simulink model "tracking_model2"  (R2017a)
settings: Solver=VariableStepAuto  StartTime=0.0  StopTime=tf  RelTol=1e-3
values from neighbouring files (symbols this model uses):
  x0 = 100    [validate_model.m]
undefined symbols (not defined in the file or in its folder): sys
settings Model: Creator=brunolnetto  LastModifiedBy=brunolnetto

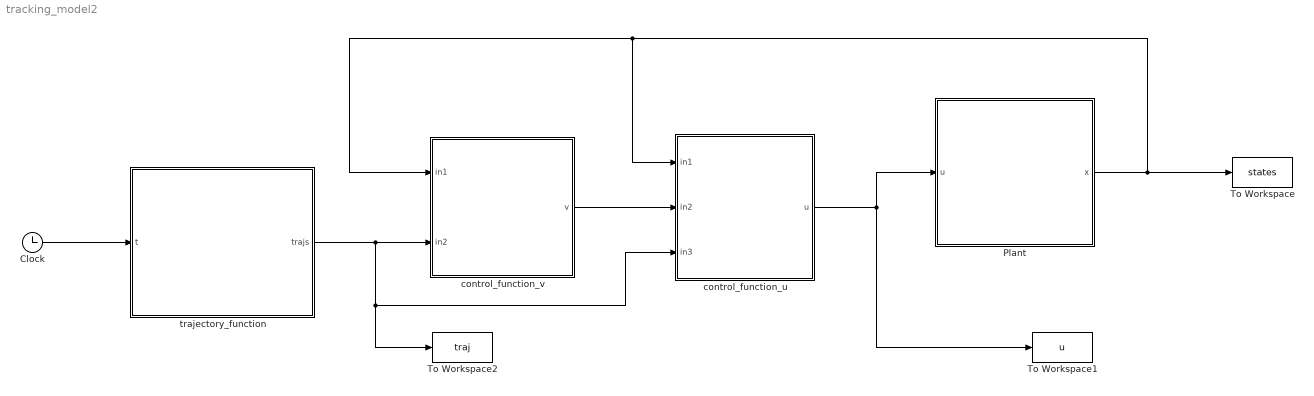
== system tracking_model2 ==
  Clock : Clock
  Plant : Subsystem
  To Workspace : ToWorkspace  VariableName=states  SaveFormat=Structure With Time  SampleTime=-1
  To Workspace1 : ToWorkspace  VariableName=u  SaveFormat=Structure With Time  SampleTime=-1
  To Workspace2 : ToWorkspace  VariableName=traj  SaveFormat=Structure With Time  SampleTime=-1
  control_function_u : MATLAB Function  TreatAsAtomicUnit=on
  control_function_v : MATLAB Function  TreatAsAtomicUnit=on
  trajectory_function : MATLAB Function  TreatAsAtomicUnit=on
  wires:
  Clock/1 -> trajectory_function/1(t)
  control_function_u/1(u) -> Plant/1(u), To Workspace1/1
  trajectory_function/1(trajs) -> control_function_u/3(in3), To Workspace2/1, control_function_v/2(in2)
  control_function_v/1(v) -> control_function_u/2(in2)
  Plant/1(x) -> control_function_u/1(in1), control_function_v/1(in1), To Workspace/1

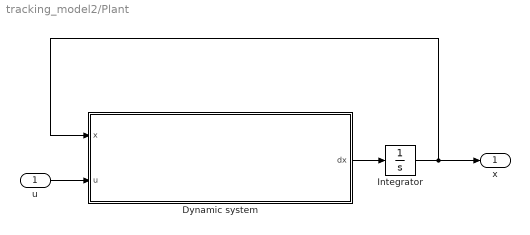
== system tracking_model2/Plant ==
  u : Inport
  Dynamic system : Subsystem
      mask Display: image('./plant.png')
  Integrator : Integrator  InitialCondition=x0
  x : Outport
  wires:
  Dynamic system/1(dx) -> Integrator/1
  u/1 -> Dynamic system/2(u)
  Integrator/1 -> x/1, Dynamic system/1(x)

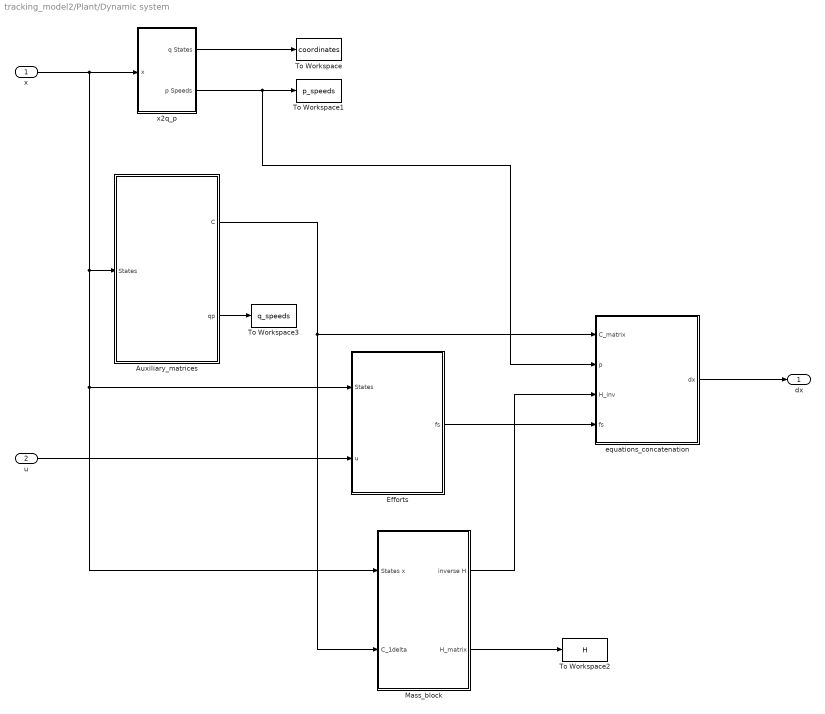
== system tracking_model2/Plant/Dynamic system ==
  x : Inport
  u : Inport  Port=2
  Auxiliary_matrices : Subsystem
  Efforts : Subsystem
  Mass_block : Subsystem
  To Workspace : ToWorkspace  VariableName=coordinates  SaveFormat=Structure With Time  SampleTime=-1
  To Workspace1 : ToWorkspace  VariableName=p_speeds  SaveFormat=Structure With Time  SampleTime=-1
  To Workspace2 : ToWorkspace  VariableName=H  SaveFormat=Structure With Time  SampleTime=-1
  To Workspace3 : ToWorkspace  VariableName=q_speeds  SaveFormat=Structure With Time  SampleTime=-1
  equations_concatenation : Subsystem
  x2q_p : Subsystem
  dx : Outport
  wires:
  Auxiliary_matrices/1(C) -> Mass_block/2("C_1delta  "), equations_concatenation/1(C_matrix)
  Auxiliary_matrices/2(qp) -> To Workspace3/1
  x2q_p/2(p Speeds) -> To Workspace1/1, equations_concatenation/2(p)
  x2q_p/1(q States) -> To Workspace/1
  Efforts/1(fs) -> equations_concatenation/4(fs)
  Mass_block/1(inverse H) -> equations_concatenation/3(H_inv)
  equations_concatenation/1(dx) -> dx/1
  u/1 -> Efforts/2(u)
  x/1 -> x2q_p/1(x), Efforts/1(States), Mass_block/1(States x), Auxiliary_matrices/1(States)
  Mass_block/2(H_matrix) -> To Workspace2/1

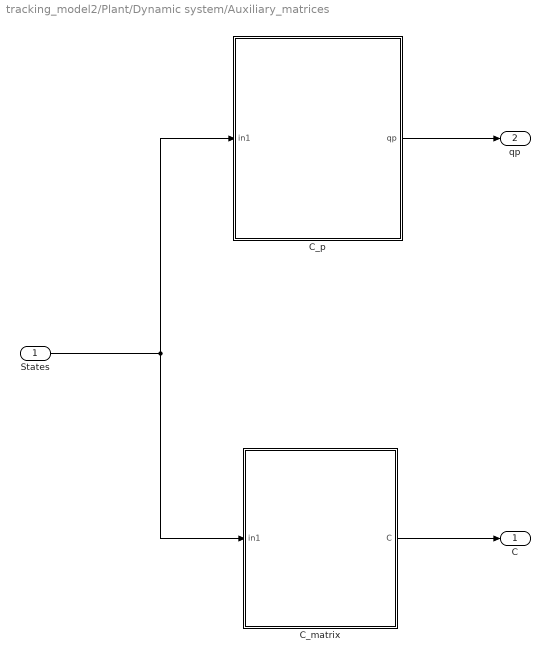
== system tracking_model2/Plant/Dynamic system/Auxiliary_matrices ==
  States : Inport
  C_matrix : MATLAB Function  TreatAsAtomicUnit=on
  C_p : MATLAB Function  TreatAsAtomicUnit=on
  C : Outport
  qp : Outport  Port=2
  wires:
  C_matrix/1(C) -> C/1
  States/1 -> C_p/1(in1), C_matrix/1(in1)
  C_p/1(qp) -> qp/1

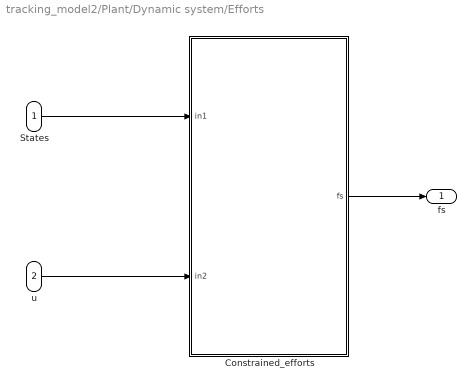
== system tracking_model2/Plant/Dynamic system/Efforts ==
  States : Inport
  u : Inport  Port=2
  Constrained_efforts : MATLAB Function  TreatAsAtomicUnit=on
  fs : Outport
  wires:
  States/1 -> Constrained_efforts/1(in1)
  u/1 -> Constrained_efforts/2(in2)
  Constrained_efforts/1(fs) -> fs/1

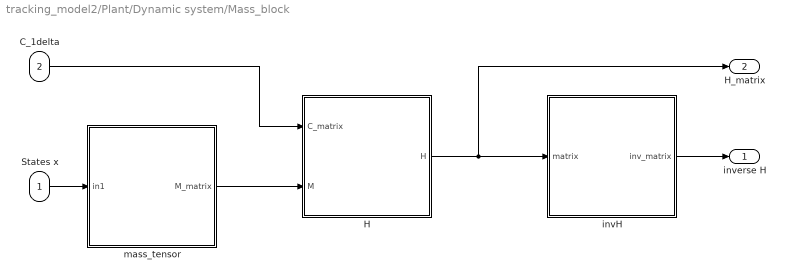
== system tracking_model2/Plant/Dynamic system/Mass_block ==
  States x : Inport
  "C_1delta  " : Inport  Port=2
  H : MATLAB Function  TreatAsAtomicUnit=on
  invH : MATLAB Function  TreatAsAtomicUnit=on
  mass_tensor : MATLAB Function  TreatAsAtomicUnit=on
  inverse H : Outport
  H_matrix : Outport  Port=2
  wires:
  States x/1 -> mass_tensor/1(in1)
  "C_1delta  "/1 -> H/1(C_matrix)
  invH/1(inv_matrix) -> inverse H/1
  H/1(H) -> invH/1(matrix), H_matrix/1
  mass_tensor/1(M_matrix) -> H/2(M)

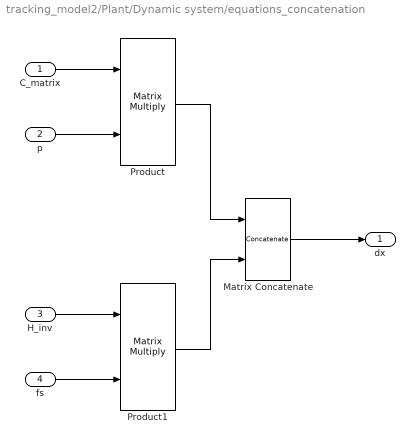
== system tracking_model2/Plant/Dynamic system/equations_concatenation ==
  C_matrix : Inport
  p : Inport  Port=2
  H_inv : Inport  Port=3
  fs : Inport  Port=4
  Matrix Concatenate : Concatenate  ConcatenateDimension=2
  Product : Product  Multiplication=Matrix(*)
  Product1 : Product  Multiplication=Matrix(*)
  dx : Outport
  wires:
  Product/1 -> Matrix Concatenate/1
  p/1 -> Product/2
  C_matrix/1 -> Product/1
  Product1/1 -> Matrix Concatenate/2
  H_inv/1 -> Product1/1
  fs/1 -> Product1/2
  Matrix Concatenate/1 -> dx/1

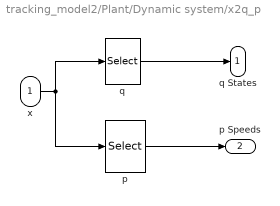
== system tracking_model2/Plant/Dynamic system/x2q_p ==
  x : Inport
  p : Selector  InputPortWidth=length(sys.kin.q) + length(sys.kin.p{end})  IndexOptions=Index vector (dialog)  Indices=(length(sys.kin.q))+1:(length(sys.kin.q) + length(sys.kin.p{end}))  OutputSizes=1
  q : Selector  InputPortWidth=length(sys.kin.q) + length(sys.kin.p{end})  IndexOptions=Index vector (dialog)  Indices=1:length(sys.kin.q)  OutputSizes=1
  q States : Outport
  p Speeds : Outport  Port=2
  wires:
  x/1 -> p/1, q/1
  q/1 -> q States/1
  p/1 -> p Speeds/1

== matlab function tracking_model2/control_function_v ==
  data: in1 input; v output; in2 input
function v = ControlFunction(in1,in2)

%    This function was generated by the Symbolic Math Toolbox version 7.2.

%    11-Jan-2021 14:43:12



p1 = in1(7,:);

p2 = in1(8,:);

p3 = in1(9,:);

th = in1(3,:);

x = in1(1,:);

y = in1(2,:);

y1_ref = in2(1,:);

y2_ref = in2(4,:);

y3_ref = in2(7,:);

yp1_ref = in2(2,:);

yp2_ref = in2(5,:);

yp3_ref = in2(8,:);

v = [p1.*-3.438624078545841-p2.*2.652700203337989-p3.*3.377020513851819e-15-th.*1.00163037277543e-14-x.*6.884313755249821-y.*1.038824780522046e1+y1_ref.*6.884313755249821+y2_ref.*1.038824780522046e1+y3_ref.*1.00163037277543e-14+yp1_ref.*3.438624078545841+yp2_ref.*2.652700203337989+yp3_ref.*3.377020513851819e-15;0.0;0.0;p1.*-2.652700278465205-p2.*7.736290108681494-p3.*1.635524904530068e-15-th.*1.056093842869619e-14-x.*1.038824829359606e1-y.*2.371441739383425e1+y1_ref.*1.038824829359606e1+y2_ref.*2.371441739383425e1+y3_ref.*1.056093842869619e-14+yp1_ref.*2.652700278465205+yp2_ref.*7.736290108681494+yp3_ref.*1.635524904530068e-15;0.0;0.0;p1.*-5.380262330691395e-15-p2.*4.786557594007766e-16-p3.*4.177097391684711-th.*6.652662314872519-x.*1.163926222557845e-14-y.*9.477276537930718e-15+y1_ref.*1.163926222557845e-14+y2_ref.*9.477276537930718e-15+y3_ref.*6.652662314872519+yp1_ref.*5.380262330691395e-15+yp2_ref.*4.786557594007766e-16+yp3_ref.*4.177097391684711;0.0;0.0];

end

== matlab function tracking_model2/Plant/Dynamic system/Mass_block/mass_tensor ==
  data: in1 input; M_matrix output
function M_matrix = Mass_matrix(in1)

%    This function was generated by the Symbolic Math Toolbox version 7.2.

%    11-Jan-2021 14:43:15



th = in1(3,:);

th1 = in1(4,:);

th2 = in1(5,:);

th3 = in1(6,:);

t2 = cos(th);

t3 = cos(th1);

t4 = cos(th2);

t5 = cos(th3);

t6 = sin(th);

t8 = t2.*(1.0./8.0);

t9 = sqrt(3.0);

t10 = t6.*t9.*(1.0./8.0);

t7 = t8-t10;

t11 = t8+t10;

t13 = t6.*(1.0./8.0);

t14 = t2.*t9.*(1.0./8.0);

t12 = t13-t14;

t15 = t13+t14;

M_matrix = reshape([2.11e2./5.0e2,0.0,0.0,0.0,0.0,0.0,0.0,2.11e2./5.0e2,0.0,0.0,0.0,0.0,0.0,0.0,t2.^2.*4.625e-3+t3.^2.*2.518133623269337e-7+t4.^2.*2.518133623269337e-7+t5.^2.*2.518133623269337e-7+t6.^2.*4.625e-3+t7.^2.*(3.7e1./5.0e2)+t11.^2.*(3.7e1./5.0e2)+t12.^2.*(3.7e1./5.0e2)+t15.^2.*(3.7e1./5.0e2)+2.520833333333333e-4,0.0,0.0,0.0,0.0,0.0,0.0,0.0,0.0,0.0,0.0,0.0,0.0,0.0,0.0,0.0,0.0,0.0,0.0,0.0,0.0,0.0],[6,6]);

end

== matlab function tracking_model2/Plant/Dynamic system/Auxiliary_matrices/C_matrix ==
  data: in1 input; C output
function C = ConstraintMatrix(in1)

%    This function was generated by the Symbolic Math Toolbox version 7.2.

%    11-Jan-2021 14:43:14



th = in1(3,:);

t2 = pi.*(1.0./3.0);

t3 = t2+th;

C = reshape([1.0,0.0,0.0,sin(th).*(5.0e2./4.3e1),cos(th+pi.*(1.0./6.0)).*(5.0e2./4.3e1),sin(t3).*(-5.0e2./4.3e1),0.0,1.0,0.0,cos(th).*(-5.0e2./4.3e1),cos(th-pi.*(1.0./3.0)).*(5.0e2./4.3e1),cos(t3).*(5.0e2./4.3e1),0.0,0.0,1.0,-1.25e2./4.3e1,-1.25e2./4.3e1,-1.25e2./4.3e1],[6,3]);

end

== matlab function tracking_model2/trajectory_function ==
  data: t input; trajs output
function trajs = TrajectoryGenerator(t)

%    This function was generated by the Symbolic Math Toolbox version 7.2.

%    11-Jan-2021 14:43:13



t2 = cos(t);

t3 = sin(t);

trajs = [t2;-t3;-t2;t3;t2;-t3;t;1.0;0.0];

end

== matlab function tracking_model2/control_function_u ==
  data: in1 input; u output; in2 input; in3 input
function u = ControlFunction(in1,in2,in3)

%    This function was generated by the Symbolic Math Toolbox version 7.2.

%    11-Jan-2021 14:43:10



p1 = in1(7,:);

p2 = in1(8,:);

p3 = in1(9,:);

th = in1(3,:);

th1 = in1(4,:);

th2 = in1(5,:);

th3 = in1(6,:);

v1 = in2(1,:);

x = in1(1,:);

y = in1(2,:);

y1_ref = in3(1,:);

y2_ref = in3(4,:);

y3_ref = in3(7,:);

yp1_ref = in3(2,:);

yp2_ref = in3(5,:);

yp3_ref = in3(8,:);

ypp1_ref = in3(3,:);

ypp2_ref = in3(6,:);

ypp3_ref = in3(9,:);

t2 = sin(th);

t3 = cos(th);

t4 = t2.^2;

t5 = t3.^2;

t6 = t5.*5.585863854409629e-2;

t7 = t4.*5.585863854409629e-2;

t8 = t6+t7;

t9 = 1.0./t8;

t10 = t5.*2.234345541763852e-1;

t11 = t4.*2.234345541763852e-1;

t12 = t10+t11;

t13 = 1.0./t12;

t14 = cos(th1);

t15 = cos(th2);

t16 = cos(th3);

t17 = t14.^2;

t18 = t15.^2;

t19 = t16.^2;

t20 = p3.^2;

t21 = t5.*5.836328869266157e-6;

t22 = t4.*5.836328869266157e-6;

t23 = t5.*t17.*1.040317779359265e-10;

t24 = t5.*t18.*1.040317779359265e-10;

t25 = t5.*t19.*1.040317779359265e-10;

t26 = t4.*t17.*1.040317779359265e-10;

t27 = t4.*t18.*1.040317779359265e-10;

t28 = t4.*t19.*1.040317779359265e-10;

t29 = t21+t22+t23+t24+t25+t26+t27+t28;

t30 = 1.0./t29;

t31 = sin(th1);

t32 = sin(th2);

t33 = sin(th3);

t34 = t31.^2;

t35 = t32.^2;

t36 = t33.^2;

t37 = th1.*2.0;

t38 = sin(t37);

t39 = th2.*2.0;

t40 = sin(t39);

t41 = th3.*2.0;

t42 = sin(t41);

t43 = t5.*1.394728536509132e-3;

t44 = t4.*1.394728536509132e-3;

t45 = t43+t44;

t46 = 1.0./t45;

t47 = p1.*p3.*t3.*t5.*t15.*t30.*t32.*t35.*-6.049843728929489e-17;

t48 = p1.*p3.*t3.*t5.*t16.*t30.*t33.*t36.*6.049843728929489e-17;

t49 = p2.*p3.*t2.*t4.*t15.*t30.*t32.*t35.*-6.049843728929489e-17;

t50 = p2.*p3.*t2.*t4.*t16.*t30.*t33.*t36.*6.049843728929489e-17;

t51 = p1.*p3.*t3.*t4.*t15.*t30.*t32.*t35.*-6.049843728929489e-17;

t52 = p1.*p3.*t3.*t5.*t15.*t30.*t32.*t34.*-6.049843728929489e-17;

t53 = p2.*p3.*t2.*t5.*t15.*t30.*t32.*t35.*-6.049843728929489e-17;

t54 = p1.*p3.*t3.*t4.*t16.*t30.*t33.*t36.*6.049843728929489e-17;

t55 = p1.*p3.*t3.*t5.*t15.*t30.*t32.*t36.*-6.049843728929489e-17;

t56 = p1.*p3.*t3.*t5.*t16.*t30.*t33.*t34.*6.049843728929489e-17;

t57 = p2.*p3.*t2.*t5.*t16.*t30.*t33.*t36.*6.049843728929489e-17;

t58 = p1.*p3.*t3.*t5.*t16.*t30.*t33.*t35.*6.049843728929489e-17;

t59 = p2.*p3.*t2.*t4.*t15.*t30.*t32.*t34.*-6.049843728929489e-17;

t60 = p2.*p3.*t2.*t4.*t15.*t30.*t32.*t36.*-6.049843728929489e-17;

t61 = p2.*p3.*t2.*t4.*t16.*t30.*t33.*t34.*6.049843728929489e-17;

t62 = p2.*p3.*t2.*t4.*t16.*t30.*t33.*t35.*6.049843728929489e-17;

t63 = p1.*p3.*t3.*t4.*t15.*t30.*t32.*t34.*-6.049843728929489e-17;

t64 = p2.*p3.*t2.*t5.*t15.*t30.*t32.*t34.*-6.049843728929489e-17;

t65 = p1.*p3.*t3.*t4.*t15.*t30.*t32.*t36.*-6.049843728929489e-17;

t66 = p1.*p3.*t3.*t4.*t16.*t30.*t33.*t34.*6.049843728929489e-17;

t67 = p1.*p3.*t3.*t4.*t16.*t30.*t33.*t35.*6.049843728929489e-17;

t68 = p2.*p3.*t2.*t5.*t15.*t30.*t32.*t36.*-6.049843728929489e-17;

t69 = p2.*p3.*t2.*t5.*t16.*t30.*t33.*t34.*6.049843728929489e-17;

t70 = p2.*p3.*t2.*t5.*t16.*t30.*t33.*t35.*6.049843728929489e-17;

t71 = p2.*t3.*t13.*-1.081184912022583e-2;

t72 = t3.*t13.*y.*-1.081184912022583e-2;

t73 = t3.*t13.*y2_ref.*1.081184912022583e-2;

t74 = t3.*t13.*yp2_ref.*1.081184912022583e-2;

t75 = t3.*t13.*ypp2_ref.*2.702962280056457e-3;

t76 = p1.*t2.*t13.*1.081184912022583e-2;

t77 = t2.*t13.*x.*1.081184912022583e-2;

t78 = t2.*t13.*y1_ref.*-1.081184912022583e-2;

t79 = t2.*t13.*yp1_ref.*-1.081184912022583e-2;

t80 = t2.*t13.*ypp1_ref.*-2.702962280056457e-3;

t81 = t5.*t20.*t30.*t34.*1.013340774614903e-53;

t82 = t5.*t20.*t30.*t35.*1.013340774614903e-53;

t83 = t5.*t20.*t30.*t36.*1.013340774614903e-53;

t84 = p3.*t5.*t9.*t34.*-6.451583127809397e-9;

t85 = p3.*t5.*t9.*t35.*-6.451583127809397e-9;

t86 = p3.*t5.*t9.*t36.*-6.451583127809397e-9;

t87 = t4.*t20.*t30.*t34.*1.013340774614903e-53;

t88 = t4.*t20.*t30.*t35.*1.013340774614903e-53;

t89 = t4.*t20.*t30.*t36.*1.013340774614903e-53;

t90 = t5.*t9.*t34.*th.*-6.451583127809397e-9;

t91 = t5.*t9.*t35.*th.*-6.451583127809397e-9;

t92 = t5.*t9.*t36.*th.*-6.451583127809397e-9;

t93 = t5.*t9.*t34.*v1.*1.612895781952349e-9;

t94 = t5.*t9.*t35.*v1.*1.612895781952349e-9;

t95 = t5.*t9.*t36.*v1.*1.612895781952349e-9;

t96 = t5.*t9.*t34.*y3_ref.*6.451583127809397e-9;

t97 = t5.*t9.*t35.*y3_ref.*6.451583127809397e-9;

t98 = t5.*t9.*t36.*y3_ref.*6.451583127809397e-9;

t99 = t5.*t9.*t34.*yp3_ref.*6.451583127809397e-9;

t100 = t5.*t9.*t35.*yp3_ref.*6.451583127809397e-9;

t101 = t5.*t9.*t36.*yp3_ref.*6.451583127809397e-9;

t102 = t5.*t9.*t34.*ypp3_ref.*1.612895781952349e-9;

t103 = t5.*t9.*t35.*ypp3_ref.*1.612895781952349e-9;

t104 = t5.*t9.*t36.*ypp3_ref.*1.612895781952349e-9;

t105 = p3.*t4.*t9.*t34.*-6.451583127809397e-9;

t106 = p3.*t4.*t9.*t35.*-6.451583127809397e-9;

t107 = p3.*t4.*t9.*t36.*-6.451583127809397e-9;

t108 = t4.*t9.*t34.*th.*-6.451583127809397e-9;

t109 = t4.*t9.*t35.*th.*-6.451583127809397e-9;

t110 = t4.*t9.*t36.*th.*-6.451583127809397e-9;

t111 = t4.*t9.*t34.*v1.*1.612895781952349e-9;

t112 = t4.*t9.*t35.*v1.*1.612895781952349e-9;

t113 = t4.*t9.*t36.*v1.*1.612895781952349e-9;

t114 = t4.*t9.*t34.*y3_ref.*6.451583127809397e-9;

t115 = t4.*t9.*t35.*y3_ref.*6.451583127809397e-9;

t116 = t4.*t9.*t36.*y3_ref.*6.451583127809397e-9;

t117 = t4.*t9.*t34.*yp3_ref.*6.451583127809397e-9;

t118 = t4.*t9.*t35.*yp3_ref.*6.451583127809397e-9;

t119 = t4.*t9.*t36.*yp3_ref.*6.451583127809397e-9;

t120 = t4.*t9.*t34.*ypp3_ref.*1.612895781952349e-9;

t121 = t4.*t9.*t35.*ypp3_ref.*1.612895781952349e-9;

t122 = t4.*t9.*t36.*ypp3_ref.*1.612895781952349e-9;

t123 = t5.*t20.*t30.*t38.*-2.449573643318391e-13;

t124 = t5.*t20.*t30.*t40.*-2.449573643318391e-13;

t125 = t5.*t20.*t30.*t42.*-2.449573643318391e-13;

t126 = t4.*t20.*t30.*t38.*-2.449573643318391e-13;

t127 = t4.*t20.*t30.*t40.*-2.449573643318391e-13;

t128 = t4.*t20.*t30.*t42.*-2.449573643318391e-13;

t129 = t5.*t20.*t30.*t34.*t38.*4.366098631815762e-18;

t130 = t5.*t20.*t30.*t35.*t38.*4.366098631815762e-18;

t131 = t5.*t20.*t30.*t34.*t40.*4.366098631815762e-18;

t132 = t5.*t20.*t30.*t36.*t38.*4.366098631815762e-18;

t133 = t5.*t20.*t30.*t35.*t40.*4.366098631815762e-18;

t134 = t5.*t20.*t30.*t34.*t42.*4.366098631815762e-18;

t135 = t5.*t20.*t30.*t36.*t40.*4.366098631815762e-18;

t136 = t5.*t20.*t30.*t35.*t42.*4.366098631815762e-18;

t137 = t5.*t20.*t30.*t36.*t42.*4.366098631815762e-18;

t138 = t4.*t20.*t30.*t34.*t38.*4.366098631815762e-18;

t139 = t4.*t20.*t30.*t35.*t38.*4.366098631815762e-18;

t140 = t4.*t20.*t30.*t34.*t40.*4.366098631815762e-18;

t141 = t4.*t20.*t30.*t36.*t38.*4.366098631815762e-18;

t142 = t4.*t20.*t30.*t35.*t40.*4.366098631815762e-18;

t143 = t4.*t20.*t30.*t34.*t42.*4.366098631815762e-18;

t144 = t4.*t20.*t30.*t36.*t40.*4.366098631815762e-18;

t145 = t4.*t20.*t30.*t35.*t42.*4.366098631815762e-18;

t146 = t4.*t20.*t30.*t36.*t42.*4.366098631815762e-18;

t147 = p2.*p3.*t3.*t5.*t14.*t30.*t31.*t34.*6.98575781090522e-17;

t148 = p2.*p3.*t3.*t5.*t15.*t30.*t32.*t35.*-3.49287890545261e-17;

t149 = p2.*p3.*t3.*t5.*t16.*t30.*t33.*t36.*-3.49287890545261e-17;

t150 = p1.*p3.*t2.*t4.*t14.*t30.*t31.*t34.*-6.98575781090522e-17;

t151 = p1.*p3.*t2.*t4.*t15.*t30.*t32.*t35.*3.49287890545261e-17;

t152 = p1.*p3.*t2.*t4.*t16.*t30.*t33.*t36.*3.49287890545261e-17;

t153 = p2.*p3.*t3.*t5.*t14.*t30.*t31.*-3.919317829309426e-12;

t154 = p1.*p3.*t3.*t5.*t15.*t30.*t32.*3.394228805687245e-12;

t155 = p2.*p3.*t3.*t5.*t15.*t30.*t32.*1.959658914654713e-12;

t156 = p1.*p3.*t3.*t5.*t16.*t30.*t33.*-3.394228805687245e-12;

t157 = p2.*p3.*t3.*t5.*t16.*t30.*t33.*1.959658914654713e-12;

t158 = p1.*p3.*t2.*t4.*t14.*t30.*t31.*3.919317829309426e-12;

t159 = p1.*p3.*t2.*t4.*t15.*t30.*t32.*-1.959658914654713e-12;

t160 = p2.*p3.*t2.*t4.*t15.*t30.*t32.*3.394228805687245e-12;

t161 = p1.*p3.*t2.*t4.*t16.*t30.*t33.*-1.959658914654713e-12;

t162 = p2.*p3.*t2.*t4.*t16.*t30.*t33.*-3.394228805687245e-12;

t163 = p1.*p3.*t2.*t5.*t14.*t30.*t31.*3.919317829309426e-12;

t164 = p2.*p3.*t3.*t4.*t14.*t30.*t31.*-3.919317829309426e-12;

t165 = p1.*p3.*t3.*t4.*t15.*t30.*t32.*3.394228805687245e-12;

t166 = p1.*p3.*t2.*t5.*t15.*t30.*t32.*-1.959658914654713e-12;

t167 = p2.*p3.*t3.*t4.*t15.*t30.*t32.*1.959658914654713e-12;

t168 = p2.*p3.*t2.*t5.*t15.*t30.*t32.*3.394228805687245e-12;

t169 = p1.*p3.*t3.*t4.*t16.*t30.*t33.*-3.394228805687245e-12;

t170 = p1.*p3.*t2.*t5.*t16.*t30.*t33.*-1.959658914654713e-12;

t171 = p2.*p3.*t3.*t4.*t16.*t30.*t33.*1.959658914654713e-12;

t172 = p2.*p3.*t2.*t5.*t16.*t30.*t33.*-3.394228805687245e-12;

t173 = p1.*p3.*t2.*t5.*t14.*t30.*t31.*t34.*-6.98575781090522e-17;

t174 = p2.*p3.*t3.*t4.*t14.*t30.*t31.*t34.*6.98575781090522e-17;

t175 = p1.*p3.*t2.*t5.*t15.*t30.*t32.*t35.*3.49287890545261e-17;

t176 = p2.*p3.*t3.*t4.*t15.*t30.*t32.*t35.*-3.49287890545261e-17;

t177 = p2.*p3.*t3.*t5.*t14.*t30.*t31.*t35.*6.98575781090522e-17;

t178 = p1.*p3.*t2.*t5.*t16.*t30.*t33.*t36.*3.49287890545261e-17;

t179 = p2.*p3.*t3.*t5.*t14.*t30.*t31.*t36.*6.98575781090522e-17;

t180 = p2.*p3.*t3.*t5.*t15.*t30.*t32.*t34.*-3.49287890545261e-17;

t181 = p2.*p3.*t3.*t4.*t16.*t30.*t33.*t36.*-3.49287890545261e-17;

t182 = p2.*p3.*t3.*t5.*t15.*t30.*t32.*t36.*-3.49287890545261e-17;

t183 = p2.*p3.*t3.*t5.*t16.*t30.*t33.*t34.*-3.49287890545261e-17;

t184 = p2.*p3.*t3.*t5.*t16.*t30.*t33.*t35.*-3.49287890545261e-17;

t185 = p1.*p3.*t2.*t4.*t14.*t30.*t31.*t35.*-6.98575781090522e-17;

t186 = p1.*p3.*t2.*t4.*t14.*t30.*t31.*t36.*-6.98575781090522e-17;

t187 = p1.*p3.*t2.*t4.*t15.*t30.*t32.*t34.*3.49287890545261e-17;

t188 = p1.*p3.*t2.*t4.*t15.*t30.*t32.*t36.*3.49287890545261e-17;

t189 = p1.*p3.*t2.*t4.*t16.*t30.*t33.*t34.*3.49287890545261e-17;

t190 = p1.*p3.*t2.*t4.*t16.*t30.*t33.*t35.*3.49287890545261e-17;

t191 = p1.*p3.*t2.*t5.*t14.*t30.*t31.*t35.*-6.98575781090522e-17;

t192 = p1.*p3.*t2.*t5.*t14.*t30.*t31.*t36.*-6.98575781090522e-17;

t193 = p1.*p3.*t2.*t5.*t15.*t30.*t32.*t34.*3.49287890545261e-17;

t194 = p2.*p3.*t3.*t4.*t14.*t30.*t31.*t35.*6.98575781090522e-17;

t195 = p2.*p3.*t3.*t4.*t14.*t30.*t31.*t36.*6.98575781090522e-17;

t196 = p2.*p3.*t3.*t4.*t15.*t30.*t32.*t34.*-3.49287890545261e-17;

t197 = p1.*p3.*t2.*t5.*t15.*t30.*t32.*t36.*3.49287890545261e-17;

t198 = p1.*p3.*t2.*t5.*t16.*t30.*t33.*t34.*3.49287890545261e-17;

t199 = p1.*p3.*t2.*t5.*t16.*t30.*t33.*t35.*3.49287890545261e-17;

t200 = p2.*p3.*t3.*t4.*t15.*t30.*t32.*t36.*-3.49287890545261e-17;

t201 = p2.*p3.*t3.*t4.*t16.*t30.*t33.*t34.*-3.49287890545261e-17;

t202 = p2.*p3.*t3.*t4.*t16.*t30.*t33.*t35.*-3.49287890545261e-17;

u = [t47+t48+t49+t50+t51+t52+t53+t54+t55+t56+t57+t58+t59+t60+t61+t62+t63+t64+t65+t66+t67+t68+t69+t70+t81+t82+t83+t84+t85+t86+t87+t88+t89+t90+t91+t92+t93+t94+t95+t96+t97+t98+t99+t100+t101+t102+t103+t104+t105+t106+t107+t108+t109+t110+t111+t112+t113+t114+t115+t116+t117+t118+t119+t120+t121+t122+t129+t130+t131+t132+t133+t134+t135+t136+t137+t138+t139+t140+t141+t142+t143+t144+t145+t146+t147+t148+t149+t150+t151+t152+t173+t174+t175+t176+t177+t178+t179+t180+t181+t182+t183+t184+t185+t186+t187+t188+t189+t190+t191+t192+t193+t194+t195+t196+t197+t198+t199+t200+t201+t202-p1.*t2.*t13.*2.162369824045165e-2+p3.*t4.*t9.*3.619622303627885e-4-p1.*t3.*t13.*5.732577381693205e-42-p2.*t2.*t13.*5.732577381693205e-42+p3.*t5.*t9.*3.619622303627885e-4+p2.*t3.*t13.*2.162369824045165e-2-t4.*t20.*t30.*5.685288085588199e-49-t5.*t20.*t30.*5.685288085588199e-49+t4.*t9.*th.*3.619622303627885e-4+t5.*t9.*th.*3.619622303627885e-4-t4.*t9.*v1.*9.049055759069713e-5-t5.*t9.*v1.*9.049055759069713e-5+t2.*t13.*v1.*5.405924560112914e-3-t3.*t13.*v1.*5.405924560112914e-3-t2.*t13.*x.*2.162369824045165e-2-t3.*t13.*x.*5.732577381693205e-42-t2.*t13.*y.*5.732577381693205e-42+t3.*t13.*y.*2.162369824045165e-2+t2.*t13.*y1_ref.*2.162369824045165e-2-t4.*t9.*y3_ref.*3.619622303627885e-4+t2.*t13.*y2_ref.*5.732577381693205e-42+t3.*t13.*y1_ref.*5.732577381693205e-42-t5.*t9.*y3_ref.*3.619622303627885e-4-t3.*t13.*y2_ref.*2.162369824045165e-2+t2.*t13.*yp1_ref.*2.162369824045165e-2-t4.*t9.*yp3_ref.*3.619622303627885e-4+t2.*t13.*yp2_ref.*5.732577381693205e-42+t3.*t13.*yp1_ref.*5.732577381693205e-42-t5.*t9.*yp3_ref.*3.619622303627885e-4-t3.*t13.*yp2_ref.*2.162369824045165e-2+t2.*t13.*ypp1_ref.*5.405924560112914e-3-t4.*t9.*ypp3_ref.*9.049055759069713e-5+t2.*t13.*ypp2_ref.*1.433144345423301e-42+t3.*t13.*ypp1_ref.*1.433144345423301e-42-t5.*t9.*ypp3_ref.*9.049055759069713e-5-t3.*t13.*ypp2_ref.*5.405924560112914e-3-t4.*t20.*t30.*t38.*2.449573643318391e-13-t5.*t20.*t30.*t38.*2.449573643318391e-13-t4.*t20.*t30.*t40.*2.449573643318391e-13-t5.*t20.*t30.*t40.*2.449573643318391e-13-t4.*t20.*t30.*t42.*2.449573643318391e-13-t5.*t20.*t30.*t42.*2.449573643318391e-13+t4.*t14.*t20.*t31.*t46.*2.341408548744586e-10+t5.*t14.*t20.*t31.*t46.*2.341408548744586e-10-t4.*t15.*t20.*t32.*t46.*1.170704274372293e-10-t5.*t15.*t20.*t32.*t46.*1.170704274372293e-10-t4.*t16.*t20.*t33.*t46.*1.170704274372293e-10-t5.*t16.*t20.*t33.*t46.*1.170704274372293e-10+p1.*p3.*t2.*t4.*t14.*t30.*t31.*3.919317829309426e-12+p1.*p3.*t2.*t5.*t14.*t30.*t31.*3.919317829309426e-12-p1.*p3.*t2.*t4.*t15.*t30.*t32.*1.959658914654713e-12-p2.*p3.*t3.*t4.*t14.*t30.*t31.*3.919317829309426e-12-p1.*p3.*t2.*t5.*t15.*t30.*t32.*1.959658914654713e-12+p1.*p3.*t3.*t4.*t15.*t30.*t32.*3.394228805687245e-12+p2.*p3.*t2.*t4.*t15.*t30.*t32.*3.394228805687245e-12-p2.*p3.*t3.*t5.*t14.*t30.*t31.*3.919317829309426e-12-p1.*p3.*t2.*t4.*t16.*t30.*t33.*1.959658914654713e-12+p1.*p3.*t3.*t5.*t15.*t30.*t32.*3.394228805687245e-12+p2.*p3.*t2.*t5.*t15.*t30.*t32.*3.394228805687245e-12+p2.*p3.*t3.*t4.*t15.*t30.*t32.*1.959658914654713e-12-p1.*p3.*t2.*t5.*t16.*t30.*t33.*1.959658914654713e-12-p1.*p3.*t3.*t4.*t16.*t30.*t33.*3.394228805687245e-12-p2.*p3.*t2.*t4.*t16.*t30.*t33.*3.394228805687245e-12+p2.*p3.*t3.*t5.*t15.*t30.*t32.*1.959658914654713e-12-p1.*p3.*t3.*t5.*t16.*t30.*t33.*3.394228805687245e-12-p2.*p3.*t2.*t5.*t16.*t30.*t33.*3.394228805687245e-12+p2.*p3.*t3.*t4.*t16.*t30.*t33.*1.959658914654713e-12+p2.*p3.*t3.*t5.*t16.*t30.*t33.*1.959658914654713e-12;t47+t48+t49+t50+t51+t52+t53+t54+t55+t56+t57+t58+t59+t60+t61+t62+t63+t64+t65+t66+t67+t68+t69+t70+t71+t72+t73+t74+t75+t76+t77+t78+t79+t80+t123+t124+t125+t126+t127+t128+t153+t154+t155+t156+t157+t158+t159+t160+t161+t162+t163+t164+t165+t166+t167+t168+t169+t170+t171+t172+p3.*t4.*t9.*3.619622303627885e-4-p1.*t3.*t13.*1.8726672e-2-p2.*t2.*t13.*1.8726672e-2+p3.*t5.*t9.*3.619622303627885e-4-t4.*t20.*t30.*5.685288085588199e-49-t5.*t20.*t30.*5.685288085588199e-49+t4.*t9.*th.*3.619622303627885e-4+t5.*t9.*th.*3.619622303627885e-4-t4.*t9.*v1.*9.049055759069713e-5-t5.*t9.*v1.*9.049055759069713e-5+t2.*t13.*v1.*1.978705719943543e-3+t3.*t13.*v1.*7.384630280056457e-3-t3.*t13.*x.*1.8726672e-2-t2.*t13.*y.*1.8726672e-2-t4.*t9.*y3_ref.*3.619622303627885e-4+t2.*t13.*y2_ref.*1.8726672e-2+t3.*t13.*y1_ref.*1.8726672e-2-t5.*t9.*y3_ref.*3.619622303627885e-4-t4.*t9.*yp3_ref.*3.619622303627885e-4+t2.*t13.*yp2_ref.*1.8726672e-2+t3.*t13.*yp1_ref.*1.8726672e-2-t5.*t9.*yp3_ref.*3.619622303627885e-4-t4.*t9.*ypp3_ref.*9.049055759069713e-5+t2.*t13.*ypp2_ref.*4.681668e-3+t3.*t13.*ypp1_ref.*4.681668e-3-t5.*t9.*ypp3_ref.*9.049055759069713e-5-p3.*t4.*t9.*t34.*6.451583127809397e-9-p3.*t4.*t9.*t35.*6.451583127809397e-9-p3.*t5.*t9.*t34.*6.451583127809397e-9-p3.*t4.*t9.*t36.*6.451583127809397e-9-p3.*t5.*t9.*t35.*6.451583127809397e-9-p3.*t5.*t9.*t36.*6.451583127809397e-9+t4.*t20.*t30.*t34.*1.013340774614903e-53+t4.*t20.*t30.*t35.*1.013340774614903e-53+t5.*t20.*t30.*t34.*1.013340774614903e-53+t4.*t20.*t30.*t36.*1.013340774614903e-53+t5.*t20.*t30.*t35.*1.013340774614903e-53+t5.*t20.*t30.*t36.*1.013340774614903e-53-t4.*t9.*t34.*th.*6.451583127809397e-9-t4.*t9.*t35.*th.*6.451583127809397e-9-t5.*t9.*t34.*th.*6.451583127809397e-9-t4.*t9.*t36.*th.*6.451583127809397e-9-t5.*t9.*t35.*th.*6.451583127809397e-9-t5.*t9.*t36.*th.*6.451583127809397e-9+t4.*t9.*t34.*v1.*1.612895781952349e-9+t4.*t9.*t35.*v1.*1.612895781952349e-9+t5.*t9.*t34.*v1.*1.612895781952349e-9+t4.*t9.*t36.*v1.*1.612895781952349e-9+t5.*t9.*t35.*v1.*1.612895781952349e-9+t5.*t9.*t36.*v1.*1.612895781952349e-9+t4.*t9.*t34.*y3_ref.*6.451583127809397e-9+t4.*t9.*t35.*y3_ref.*6.451583127809397e-9+t5.*t9.*t34.*y3_ref.*6.451583127809397e-9+t4.*t9.*t36.*y3_ref.*6.451583127809397e-9+t5.*t9.*t35.*y3_ref.*6.451583127809397e-9+t5.*t9.*t36.*y3_ref.*6.451583127809397e-9+t4.*t9.*t34.*yp3_ref.*6.451583127809397e-9+t4.*t9.*t35.*yp3_ref.*6.451583127809397e-9+t5.*t9.*t34.*yp3_ref.*6.451583127809397e-9+t4.*t9.*t36.*yp3_ref.*6.451583127809397e-9+t5.*t9.*t35.*yp3_ref.*6.451583127809397e-9+t5.*t9.*t36.*yp3_ref.*6.451583127809397e-9+t4.*t9.*t34.*ypp3_ref.*1.612895781952349e-9+t4.*t9.*t35.*ypp3_ref.*1.612895781952349e-9+t5.*t9.*t34.*ypp3_ref.*1.612895781952349e-9+t4.*t9.*t36.*ypp3_ref.*1.612895781952349e-9+t5.*t9.*t35.*ypp3_ref.*1.612895781952349e-9+t5.*t9.*t36.*ypp3_ref.*1.612895781952349e-9-t4.*t14.*t20.*t31.*t46.*1.170704274372293e-10-t5.*t14.*t20.*t31.*t46.*1.170704274372293e-10+t4.*t15.*t20.*t32.*t46.*2.341408548744586e-10+t5.*t15.*t20.*t32.*t46.*2.341408548744586e-10-t4.*t16.*t20.*t33.*t46.*1.170704274372293e-10-t5.*t16.*t20.*t33.*t46.*1.170704274372293e-10+t4.*t20.*t30.*t34.*t38.*4.366098631815762e-18+t4.*t20.*t30.*t35.*t38.*4.366098631815762e-18+t5.*t20.*t30.*t34.*t38.*4.366098631815762e-18+t4.*t20.*t30.*t34.*t40.*4.366098631815762e-18+t4.*t20.*t30.*t36.*t38.*4.366098631815762e-18+t5.*t20.*t30.*t35.*t38.*4.366098631815762e-18+t4.*t20.*t30.*t35.*t40.*4.366098631815762e-18+t5.*t20.*t30.*t34.*t40.*4.366098631815762e-18+t5.*t20.*t30.*t36.*t38.*4.366098631815762e-18+t4.*t20.*t30.*t34.*t42.*4.366098631815762e-18+t4.*t20.*t30.*t36.*t40.*4.366098631815762e-18+t5.*t20.*t30.*t35.*t40.*4.366098631815762e-18+t4.*t20.*t30.*t35.*t42.*4.366098631815762e-18+t5.*t20.*t30.*t34.*t42.*4.366098631815762e-18+t5.*t20.*t30.*t36.*t40.*4.366098631815762e-18+t4.*t20.*t30.*t36.*t42.*4.366098631815762e-18+t5.*t20.*t30.*t35.*t42.*4.366098631815762e-18+t5.*t20.*t30.*t36.*t42.*4.366098631815762e-18-p1.*p3.*t2.*t4.*t14.*t30.*t31.*t34.*6.98575781090522e-17-p1.*p3.*t2.*t4.*t14.*t30.*t31.*t35.*6.98575781090522e-17-p1.*p3.*t2.*t5.*t14.*t30.*t31.*t34.*6.98575781090522e-17-p1.*p3.*t2.*t4.*t14.*t30.*t31.*t36.*6.98575781090522e-17+p1.*p3.*t2.*t4.*t15.*t30.*t32.*t34.*3.49287890545261e-17-p1.*p3.*t2.*t5.*t14.*t30.*t31.*t35.*6.98575781090522e-17+p2.*p3.*t3.*t4.*t14.*t30.*t31.*t34.*6.98575781090522e-17+p1.*p3.*t2.*t4.*t15.*t30.*t32.*t35.*3.49287890545261e-17-p1.*p3.*t2.*t5.*t14.*t30.*t31.*t36.*6.98575781090522e-17+p1.*p3.*t2.*t5.*t15.*t30.*t32.*t34.*3.49287890545261e-17+p2.*p3.*t3.*t4.*t14.*t30.*t31.*t35.*6.98575781090522e-17+p2.*p3.*t3.*t5.*t14.*t30.*t31.*t34.*6.98575781090522e-17+p1.*p3.*t2.*t4.*t15.*t30.*t32.*t36.*3.49287890545261e-17+p1.*p3.*t2.*t4.*t16.*t30.*t33.*t34.*3.49287890545261e-17+p1.*p3.*t2.*t5.*t15.*t30.*t32.*t35.*3.49287890545261e-17+p2.*p3.*t3.*t4.*t14.*t30.*t31.*t36.*6.98575781090522e-17-p2.*p3.*t3.*t4.*t15.*t30.*t32.*t34.*3.49287890545261e-17+p2.*p3.*t3.*t5.*t14.*t30.*t31.*t35.*6.98575781090522e-17+p1.*p3.*t2.*t4.*t16.*t30.*t33.*t35.*3.49287890545261e-17+p1.*p3.*t2.*t5.*t15.*t30.*t32.*t36.*3.49287890545261e-17+p1.*p3.*t2.*t5.*t16.*t30.*t33.*t34.*3.49287890545261e-17-p2.*p3.*t3.*t4.*t15.*t30.*t32.*t35.*3.49287890545261e-17+p2.*p3.*t3.*t5.*t14.*t30.*t31.*t36.*6.98575781090522e-17-p2.*p3.*t3.*t5.*t15.*t30.*t32.*t34.*3.49287890545261e-17+p1.*p3.*t2.*t4.*t16.*t30.*t33.*t36.*3.49287890545261e-17+p1.*p3.*t2.*t5.*t16.*t30.*t33.*t35.*3.49287890545261e-17-p2.*p3.*t3.*t4.*t15.*t30.*t32.*t36.*3.49287890545261e-17-p2.*p3.*t3.*t4.*t16.*t30.*t33.*t34.*3.49287890545261e-17-p2.*p3.*t3.*t5.*t15.*t30.*t32.*t35.*3.49287890545261e-17+p1.*p3.*t2.*t5.*t16.*t30.*t33.*t36.*3.49287890545261e-17-p2.*p3.*t3.*t4.*t16.*t30.*t33.*t35.*3.49287890545261e-17-p2.*p3.*t3.*t5.*t15.*t30.*t32.*t36.*3.49287890545261e-17-p2.*p3.*t3.*t5.*t16.*t30.*t33.*t34.*3.49287890545261e-17-p2.*p3.*t3.*t4.*t16.*t30.*t33.*t36.*3.49287890545261e-17-p2.*p3.*t3.*t5.*t16.*t30.*t33.*t35.*3.49287890545261e-17-p2.*p3.*t3.*t5.*t16.*t30.*t33.*t36.*3.49287890545261e-17;t47+t48+t49+t50+t51+t52+t53+t54+t55+t56+t57+t58+t59+t60+t61+t62+t63+t64+t65+t66+t67+t68+t69+t70+t71+t72+t73+t74+t75+t76+t77+t78+t79+t80+t81+t82+t83+t84+t85+t86+t87+t88+t89+t90+t91+t92+t93+t94+t95+t96+t97+t98+t99+t100+t101+t102+t103+t104+t105+t106+t107+t108+t109+t110+t111+t112+t113+t114+t115+t116+t117+t118+t119+t120+t121+t122+t123+t124+t125+t126+t127+t128+t129+t130+t131+t132+t133+t134+t135+t136+t137+t138+t139+t140+t141+t142+t143+t144+t145+t146+t147+t148+t149+t150+t151+t152+t153+t154+t155+t156+t157+t158+t159+t160+t161+t162+t163+t164+t165+t166+t167+t168+t169+t170+t171+t172+t173+t174+t175+t176+t177+t178+t179+t180+t181+t182+t183+t184+t185+t186+t187+t188+t189+t190+t191+t192+t193+t194+t195+t196+t197+t198+t199+t200+t201+t202+p3.*t4.*t9.*3.619622303627885e-4+p1.*t3.*t13.*1.8726672e-2+p2.*t2.*t13.*1.8726672e-2+p3.*t5.*t9.*3.619622303627885e-4-t4.*t20.*t30.*5.685288085588199e-49-t5.*t20.*t30.*5.685288085588199e-49+t4.*t9.*th.*3.619622303627885e-4+t5.*t9.*th.*3.619622303627885e-4-t4.*t9.*v1.*9.049055759069713e-5-t5.*t9.*v1.*9.049055759069713e-5-t2.*t13.*v1.*7.384630280056457e-3-t3.*t13.*v1.*1.978705719943543e-3+t3.*t13.*x.*1.8726672e-2+t2.*t13.*y.*1.8726672e-2-t4.*t9.*y3_ref.*3.619622303627885e-4-t2.*t13.*y2_ref.*1.8726672e-2-t3.*t13.*y1_ref.*1.8726672e-2-t5.*t9.*y3_ref.*3.619622303627885e-4-t4.*t9.*yp3_ref.*3.619622303627885e-4-t2.*t13.*yp2_ref.*1.8726672e-2-t3.*t13.*yp1_ref.*1.8726672e-2-t5.*t9.*yp3_ref.*3.619622303627885e-4-t4.*t9.*ypp3_ref.*9.049055759069713e-5-t2.*t13.*ypp2_ref.*4.681668e-3-t3.*t13.*ypp1_ref.*4.681668e-3-t5.*t9.*ypp3_ref.*9.049055759069713e-5-t4.*t14.*t20.*t31.*t46.*1.170704274372293e-10-t5.*t14.*t20.*t31.*t46.*1.170704274372293e-10-t4.*t15.*t20.*t32.*t46.*1.170704274372293e-10-t5.*t15.*t20.*t32.*t46.*1.170704274372293e-10+t4.*t16.*t20.*t33.*t46.*2.341408548744586e-10+t5.*t16.*t20.*t33.*t46.*2.341408548744586e-10];

end

== matlab function tracking_model2/Plant/Dynamic system/Efforts/Constrained_efforts ==
  data: in1 input; fs output; in2 input
function fs = ConstrainedEffort(in1,in2)

%    This function was generated by the Symbolic Math Toolbox version 7.2.

%    11-Jan-2021 14:43:15



p1 = in1(7,:);

p2 = in1(8,:);

p3 = in1(9,:);

tau1 = in2(1,:);

tau2 = in2(2,:);

tau3 = in2(3,:);

th = in1(3,:);

th1 = in1(4,:);

th2 = in1(5,:);

th3 = in1(6,:);

t2 = sin(th);

t3 = sqrt(3.0);

t4 = cos(th);

t5 = p3.^2;

t6 = t2.*t3;

t7 = cos(th2);

t8 = sin(th2);

t9 = th+1.047197551196598;

t10 = cos(th3);

t11 = sin(th3);

t12 = cos(th1);

t13 = sin(th1);

t14 = p3.*t2.*1.25e-1;

t36 = p3.*t4.*2.165063509461097e-1;

t35 = -t36;

t33 = -t35;

t28 = -t33;

t17 = -t28;

t15 = -t17;

t16 = t14+t15;

t18 = t4.*1.25e-1;

t37 = p3.*t4.*-1.25e-1;

t31 = -t37;

t30 = -t31;

t19 = -t30;

t34 = p3.*t2.*2.165063509461097e-1;

t32 = -t34;

t20 = -t32;

t21 = t4.*2.165063509461097e-1;

t22 = p2.*-1.0;

t23 = t19+t20+t22;

t24 = t2.*1.25e-1;

t25 = t21-t24;

t26 = t2.*2.165063509461097e-1;

t27 = t18+t26;

t29 = t21+t24;

t38 = p3.*t4.*(1.0./4.0);

t39 = p2+t38;

t40 = p3.*t2.*-2.5e-1;

t41 = p1+t40;

t42 = th+5.235987755982989e-1;

t43 = cos(t42);

t44 = th-1.047197551196598;

t45 = cos(t44);

t46 = p3.*(1.25e2./4.3e1);

t47 = cos(t9);

t48 = sin(t9);

fs = [t2.*tau1.*(5.0e2./4.3e1)-tau2.*(t2-t3.*t4).*(2.5e2./4.3e1)-tau3.*(t2+t3.*t4).*(2.5e2./4.3e1)-t2.*t5.*t12.*t13.*2.928062352638764e-6-t5.*t7.*t8.*t43.*2.928062352638764e-6+t5.*t10.*t11.*t48.*2.928062352638764e-6;tau2.*(t4+t6).*(2.5e2./4.3e1)-t4.*tau1.*(5.0e2./4.3e1)+tau3.*(t4-t6).*(2.5e2./4.3e1)+t4.*t5.*t12.*t13.*2.928062352638764e-6-t5.*t7.*t8.*t45.*2.928062352638764e-6-t5.*t10.*t11.*t47.*2.928062352638764e-6;tau1.*(-1.25e2./4.3e1)-tau2.*(1.25e2./4.3e1)-tau3.*(1.25e2./4.3e1)-t16.*t23.*(3.7e1./5.0e2)+p3.*(t25.*(t19+t20).*7.4e-2+t2.*t39.*1.85e-2+t16.*t27.*(3.7e1./5.0e2)+t4.*t41.*1.85e-2-t23.*t25.*(3.7e1./5.0e2)+(t14+t17).*(t18-t26).*(3.7e1./5.0e2)-t29.*(t19-p3.*t2.*2.165063509461097e-1).*7.4e-2-t27.*(p1+t14+t28).*7.4e-2-t29.*(p2+t20+t30).*7.4e-2-(t18-t26).*(p1+t14+t17).*7.4e-2).*1.0+(t31+t32).*(p1+t14+t33).*7.4e-2+(t31+t34).*(p1+t14+t35).*7.4e-2+(t14+t36).*(p2+t34+t37).*7.4e-2-p3.*t2.*t39.*1.85e-2-p3.*t4.*t41.*1.85e-2+t5.*t7.*t8.*7.32015588159691e-7+t5.*t10.*t11.*7.32015588159691e-7+t5.*t12.*t13.*7.32015588159691e-7-p3.*t12.*t13.*(t46-p1.*t2.*1.162790697674419e1+p2.*t4.*(5.0e2./4.3e1)).*5.036267246538674e-7-p3.*t10.*t11.*(t46+p1.*t48.*(5.0e2./4.3e1)-p2.*t47.*1.162790697674419e1).*5.036267246538674e-7+p3.*t7.*t8.*(p3.*-2.906976744186047+p1.*t43.*(5.0e2./4.3e1)+p2.*t45.*(5.0e2./4.3e1)).*5.036267246538674e-7];

end

== matlab function tracking_model2/Plant/Dynamic system/Mass_block/H ==
  data: C_matrix input; H output; M input
function H = ConstrinedMassMatrix(C_matrix, M)
% MASSMATRIX
%    This function was generated by the Symbolic Math Toolbox version 7.2.
%    16-Oct-2020 11:55:07

    H = C_matrix'*M*C_matrix;
end

== matlab function tracking_model2/Plant/Dynamic system/Mass_block/invH ==
  data: matrix input; inv_matrix output
function inv_matrix = matrix_inverse(matrix)
% MASSMATRIX
%    This function was generated by the Symbolic Math Toolbox version 7.2.
%    16-Oct-2020 11:55:07

    inv_matrix = inv(matrix);
end

== matlab function tracking_model2/Plant/Dynamic system/Auxiliary_matrices/C_p ==
  data: in1 input; qp output
function qp = KinematicVector(in1)

%    This function was generated by the Symbolic Math Toolbox version 7.2.

%    11-Jan-2021 14:43:14



p1 = in1(7,:);

p2 = in1(8,:);

p3 = in1(9,:);

th = in1(3,:);

t2 = pi.*(1.0./3.0);

t3 = t2+th;

qp = [p1;p2;p3;p3.*(-1.25e2./4.3e1)-p2.*cos(th).*(5.0e2./4.3e1)+p1.*sin(th).*(5.0e2./4.3e1);p3.*(-1.25e2./4.3e1)+p2.*cos(th-pi.*(1.0./3.0)).*(5.0e2./4.3e1)+p1.*cos(th+pi.*(1.0./6.0)).*(5.0e2./4.3e1);p3.*(-1.25e2./4.3e1)+p2.*cos(t3).*(5.0e2./4.3e1)-p1.*sin(t3).*(5.0e2./4.3e1)];

end
